simulink model "drive_impl"  (R2021a)
settings: Solver=ode23s  StartTime=0.0  StopTime=5  FixedStep=1e-4  MaxStep=1e-3  RelTol=1e-3  EnableMultiTasking=on
InitFcn:
  | run('balancing_in_one_place_code.m');
values from neighbouring files (symbols this model uses):
  Cm = Ce    (= 0.0527)    [drive_params.m]
  h_val = R*2    (= 0.228)    [drive_imp_code.m]
  J_rolik = 1/4*m_rolik*r_val^2 + 1/12*m_rolik*h_val^2    [Initial_code.m]    (also in drive_imp_code.m = 4.5350625e-08)
  J_sphere = 2*M*R^2/5    (= 0.0038988)    [Initial_code.m]    (also in drive_imp_code.m)
  K_reg = place(A,B,p)    [Initial_code.m]    (also in drive_imp_code.m)
  Kconv = Udc    [drive_params.m]
  Kfb_i = 1/In    [drive_params.m]
  Ki = Te/(2*Kfb_i*(1/Cma)*Tconv*Kconv/Cea*b)    [drive_params.m]
  Klship = 1    [drive_params.m]
  L = 0.3    [Initial_code.m]    (also in drive_imp_code.m = 0.5)
  lenght_rolik = R+r_val    (= 0.1425)    [Initial_code.m]    (also in drive_imp_code.m)
  m = 1.5    [Initial_code.m]    (also in drive_imp_code.m)
  M = 0.75    [Initial_code.m]    (also in drive_imp_code.m)
  m_rolik = 1e-5    (= 1e-05)    [Initial_code.m]    (also in drive_imp_code.m)
  R = 0.114    [Initial_code.m]    (also in drive_imp_code.m)
  r_val = R*0.25    (= 0.0285)    [Initial_code.m]    (also in drive_imp_code.m)
  T = Tk    (= 1e-05)    [drive_params.m]
  Tconv = 0.5*T    (= 5e-06)    [drive_params.m]
  Ti = Te    (= 0.000136363636364)    [drive_params.m]
  U_nom = 12    [drive_params.m]
undefined symbols (not defined in the file or in its folder): DiscIntNeverNeededParam, X, Y, Z
libraries: sm_lib x87, nesl_utility x32, fl_lib x23, simulink x10, fl_ps_legacy_lib x9, ee_lib x8, simulink_extras x4, pid_lib x1
(part 1 of 4)
settings Model: Creator=fawnt  LastModifiedBy=Rita-Margarita
settings SolverCC: ZeroCrossAlgorithm=Adaptive  AlgebraicLoopSolver=TrustRegion
settings DataIOCC: LimitDataPoints=on  SaveFormat=Array
settings OptimizationCC: LifeSpan=inf
settings DebuggingCC: IgnoredZcDiagnostic=none  SolverPrmCheckMsg=warning  OperatingPointInterfaceChecksumMismatchMsg=none  SFUnexpectedBacktrackingDiag=warning  SFNoUnconditionalDefaultTransitionDiag=warning  SFExecutionAtInitializationDiag=none  SFMachineParentedDataDiag=warning  ArithmeticOperatorsInVariantConditions=warning
settings HardwareCC: ProdBitPerPointer=32  ProdBitPerSizeT=32  ProdBitPerPtrDiffT=32  ProdLargestAtomicFloat=None  ProdIntDivRoundTo=Undefined  ProdEndianess=Unspecified  ProdWordSize=32  ProdHWDeviceType=32-bit Generic
settings ModelReferenceCC: PropagateSignalLabelsOutOfModel=off
settings SFSimCC: SimUseLocalCustomCode=off  CustomCodeUndefinedFunction=UseInterfaceOnly
settings RTWCC: RTWUseLocalCustomCode=off
settings CodeAppCC: StateflowObjectComments=on
settings GRTTargetCC: TargetLangStandard=C89/C90 (ANSI)
settings ConfigComp: CovMetricSettings=dw  CovSaveCumulativeToWorkspaceVar=on  CovSaveSingleToWorkspaceVar=on  CovExternalEMLEnable=off  CovSFcnEnable=off
settings SimscapeCC: SimscapeNormalizeSystem=off
settings ConfigurationSet: Description=SimMechanics 2G
settings DiagnosticsConfigSet: SimMechanicsRigidlyBoundBlock=none
settings ExplorerConfigSet: InternalSimMechanicsExplorerSettings="<ExplorerConfiguration><canonicalview>default</canonicalview><AnimationSetting><BasePlaybackSpeed>1.0</BasePlaybackSpeed><PlaybackSpeedFactor>1.0</PlaybackSpeedFactor></AnimationSetting><TilePanel><TileInfo><Tiles Columns=\"1\" Count=\"1\" Rows=\"1\"><Column Weight=\"1\"/><Row Weight=\"1\"/><Tile Height=\"1\" Width=\"1\" X=\"0\" Y=\"0\"/></Tiles></TileInfo><SceneInfo><SceneViewer><BGColor><R>1</R><G>1</G><B>1</B></BGColor><Camera><DoPerspective>off</DoPerspective><Position><X>0.176630985411527358</X><Y>-21.2723354631550592</Y><Z>0.23862415286042904</Z></Position><Center><X>0.176630985411527358</X><Y>8.40499914944725646e-07</Y><Z>0.23862415286042904</Z></Center><Up><X>0</X><Y>-0</Y><Z>1</Z></Up><ViewLimDist>1</ViewLimDist><YLim>0.435658064716423932</YLim><XLim>0.654723357190176269</XLim></Camera></SceneViewer></SceneInfo></TilePanel><MechEditorPanel><Cameras/><GfxPanelCameraMap/><VideoCreator><PlaybackSpeedRatio>1.0</PlaybackSpeedRatio><FrameRate>30</FrameRate><VideoFormat>Motion JPEG 2000</VideoFormat><FrameSize>auto</FrameSize></VideoCreator></MechEditorPanel></ExplorerConfiguration>"

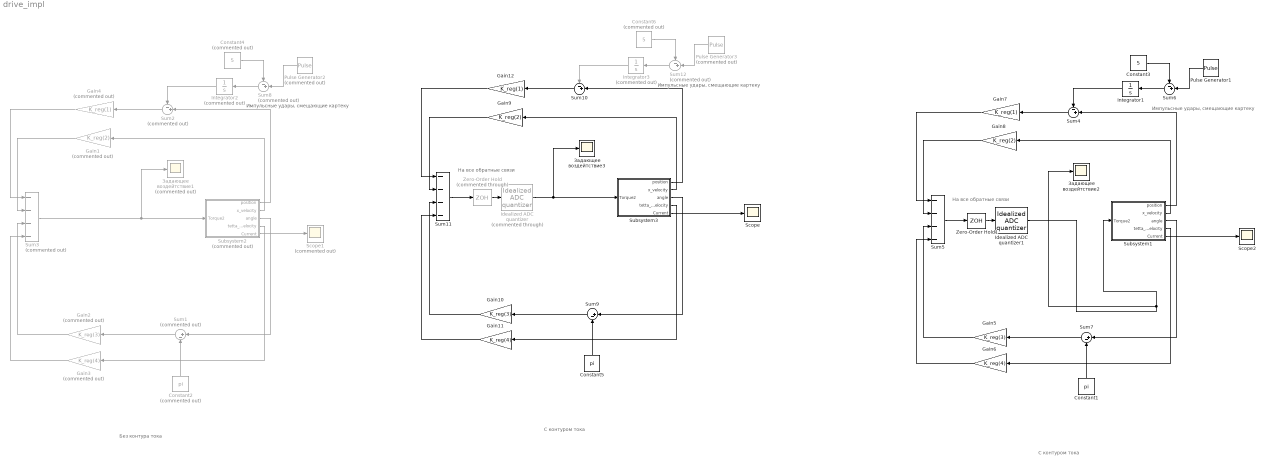
== system drive_impl ==
  note: Без контура тока
  note: Импульсные удары, смещающие картеку
  note: Импульсные удары, смещающие картеку
  note: С контуром тока
  note: На все обратные связи
  note: Импульсные удары, смещающие картеку
  note: С контуром тока
  note: На все обратные связи
  Constant1 : Constant  Value=pi
  Constant2 : Constant  Commented=on  Value=pi
  Constant3 : Constant  Value=5
  Constant4 : Constant  Commented=on  Value=5
  Constant5 : Constant  Value=pi
  Constant6 : Constant  Commented=on  Value=5
  Gain1 : Gain  Commented=on  Gain=K_reg(2)
  Gain10 : Gain  Gain=K_reg(3)
  Gain11 : Gain  Gain=K_reg(4)
  Gain12 : Gain  Gain=K_reg(1)
  Gain2 : Gain  Commented=on  Gain=K_reg(3)
  Gain3 : Gain  Commented=on  Gain=K_reg(4)
  Gain4 : Gain  Commented=on  Gain=K_reg(1)
  Gain5 : Gain  Gain=K_reg(3)
  Gain6 : Gain  Gain=K_reg(4)
  Gain7 : Gain  Gain=K_reg(1)
  Gain8 : Gain  Gain=K_reg(2)
  Gain9 : Gain  Gain=K_reg(2)
  Idealized ADC quantizer : simulink_extras/Additional Discrete/Idealized ADC quantizer  Commented=through  NumberOfConverterBits=12  Vmin=0  Vmax=12  OutputDataType=int16  OutputNegativeValues=on
  Idealized ADC quantizer1 : simulink_extras/Additional Discrete/Idealized ADC quantizer  NumberOfConverterBits=12  Vmin=0  Vmax=12  OutputDataType=int16  OutputNegativeValues=on
  Integrator1 : Integrator  LimitOutput=on  UpperSaturationLimit=10  LowerSaturationLimit=-10
  Integrator2 : Integrator  Commented=on  LimitOutput=on  UpperSaturationLimit=3  LowerSaturationLimit=-3
  Integrator3 : Integrator  Commented=on  LimitOutput=on  UpperSaturationLimit=10  LowerSaturationLimit=-10
  Pulse Generator1 : DiscretePulseGenerator  PulseType=Time based  Amplitude=10  Period=10  PulseWidth=50
  Pulse Generator2 : DiscretePulseGenerator  Commented=on  PulseType=Time based  Amplitude=10  Period=10  PulseWidth=50
  Pulse Generator3 : DiscretePulseGenerator  Commented=on  PulseType=Time based  Amplitude=10  Period=10  PulseWidth=50
  Scope : Scope
  Scope1 : Scope  Commented=on
  Scope2 : Scope
  Subsystem1 : Subsystem
  Subsystem2 : Subsystem  Commented=on
  Subsystem3 : Subsystem
  Sum1 : Sum  Commented=on  Inputs=|+-
  Sum10 : Sum  Inputs=-+|
  Sum11 : Sum  Inputs=----
  Sum12 : Sum  Commented=on  Inputs=-+|
  Sum2 : Sum  Commented=on  Inputs=-+|
  Sum3 : Sum  Commented=on  Inputs=----
  Sum4 : Sum  Inputs=-+|
  Sum5 : Sum  Inputs=----
  Sum6 : Sum  Inputs=-+|
  Sum7 : Sum  Inputs=|+-
  Sum8 : Sum  Commented=on  Inputs=-+|
  Sum9 : Sum  Inputs=|+-
  Zero-Order Hold : ZeroOrderHold  Commented=through  SampleTime=1/(20e3)
  Zero-Order Hold1 : ZeroOrderHold  SampleTime=1/(20e3)
  Задающее воздейтствие1 : Scope  Commented=on
  Задающее воздейтствие2 : Scope
  Задающее воздейтствие3 : Scope
  wires:
  Gain2/1 -> Sum3/3
  Constant2/1 -> Sum1/2
  Subsystem2/4("tetta_velocity ") -> Gain3/1
  Sum2/1 -> Gain4/1
  Integrator2/1 -> Sum2/1
  Gain3/1 -> Sum3/4
  Sum3/1 -> Задающее воздейтствие1/1, Subsystem2/1(Torque2)
  Sum8/1 -> Integrator2/1
  Subsystem2/1(position) -> Sum2/2
  Subsystem2/3(angle) -> Sum1/1
  Gain4/1 -> Sum3/1
  Constant4/1 -> Sum8/1
  Subsystem2/2("x_velocity ") -> Gain1/1
  Pulse Generator2/1 -> Sum8/2
  Gain1/1 -> Sum3/2
  Sum1/1 -> Gain2/1
  Subsystem3/4("tetta_velocity ") -> Gain11/1
  Pulse Generator3/1 -> Sum12/2
  Sum10/1 -> Gain12/1
  Subsystem3/1(position) -> Sum10/2
  Gain10/1 -> Sum11/3
  Constant6/1 -> Sum12/1
  Integrator3/1 -> Sum10/1
  Subsystem3/3(angle) -> Sum9/1
  Gain11/1 -> Sum11/4
  Constant5/1 -> Sum9/2
  Subsystem3/2("x_velocity ") -> Gain9/1
  Sum11/1 -> Zero-Order Hold/1
  Gain12/1 -> Sum11/1
  Sum12/1 -> Integrator3/1
  Sum9/1 -> Gain10/1
  Gain9/1 -> Sum11/2
  Subsystem3/5(Current) -> Scope/1
  Subsystem2/5(Current) -> Scope1/1
  Zero-Order Hold/1 -> Idealized ADC quantizer/1
  Idealized ADC quantizer/1 -> Subsystem3/1(Torque2), Задающее воздейтствие3/1
  Subsystem1/5(Current) -> Scope2/1
  Subsystem1/4("tetta_velocity ") -> Gain6/1
  Pulse Generator1/1 -> Sum6/2
  Sum6/1 -> Integrator1/1
  Gain7/1 -> Sum5/1
  Gain6/1 -> Sum5/4
  Sum4/1 -> Gain7/1
  Constant1/1 -> Sum7/2
  Subsystem1/1(position) -> Sum4/2
  Sum5/1 -> Zero-Order Hold1/1
  Constant3/1 -> Sum6/1
  Integrator1/1 -> Sum4/1
  Idealized ADC quantizer1/1 -> Subsystem1/1(Torque2), Задающее воздейтствие2/1
  Sum7/1 -> Gain5/1
  Gain5/1 -> Sum5/3
  Subsystem1/2("x_velocity ") -> Gain8/1
  Subsystem1/3(angle) -> Sum7/1
  Gain8/1 -> Sum5/2
  Zero-Order Hold1/1 -> Idealized ADC quantizer1/1
